simulink model "MPC_System"  (R2019a)
settings: Solver=VariableStepAuto  StartTime=0.0  StopTime=20  RelTol=1e-3
libraries: sailbot_library x19, mpclib x1
settings Model: Creator=ronak  LastModifiedBy=brucecui
settings DataIOCC: SaveFormat=StructureWithTime

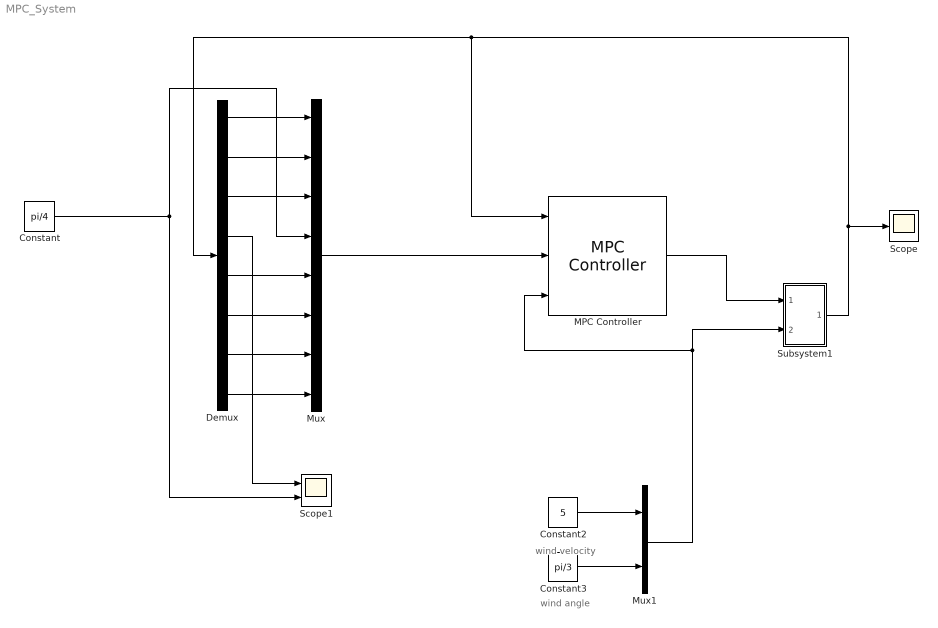
== system MPC_System ==
  note: wind velocity
  note: wind angle
  Constant : Constant  Value=pi/4
  Constant2 : Constant  Value=5
  Constant3 : Constant  Value=pi/3
  Demux : Demux  Outputs=8
  MPC Controller : mpclib/MPC Controller  SCDEnableBlockLinearizationSpecification=on  mpcobj=mpc1  is_multiple=0  enable_value=0  return_u0=off  updateMPCinCallerWorkspace=on  md_inport=on  mv_inport=off  uref_inport=off  return_cost=off  return_mvseq=off  return_qpstatus=off  return_xseq=off  return_state=off  return_ovseq=off  state_inport=off  umin_inport=off  umax_inport=off  ymin_inport=off  ymax_inport=off  cc_inport=off  ywt_inport=off  uwt_inport=off  duwt_inport=off  rhoeps_inport=off  pm_inport=off  MaximumP=10  HorizonChoice=FixedHorizon  n_ts=1  n_p=10  n_mv=2  n_md=2  n_ud=0  n_mo=8  n_uo=0  BlockDataType=double  SampleTimeInherited=off  switch_inport=off
      settings: SourceProductName=MATLAB Runtime - Model Predictive Control Toolbox Addin  SourceProductBaseCode=Missing
  Mux : Mux  Inputs=8
  Mux1 : Mux  Inputs=2
  Scope : Scope
  Scope1 : Scope  NumInputPorts=2
  Subsystem1 : Subsystem
  wires:
  Constant2/1 -> Mux1/1
  Demux/1 -> Mux/1
  Demux/2 -> Mux/2
  Demux/7 -> Mux/7
  Demux/3 -> Mux/3
  MPC Controller/1 -> Subsystem1/1(In1)
  Demux/8 -> Mux/8
  Demux/5 -> Mux/5
  Constant/1 -> Scope1/2, Mux/4
  Constant3/1 -> Mux1/2
  Demux/4 -> Scope1/1
  Demux/6 -> Mux/6
  Mux/1 -> MPC Controller/2
  Subsystem1/1(Out2) -> Scope/1, MPC Controller/1, Demux/1
  Mux1/1 -> MPC Controller/3, Subsystem1/2(In2)

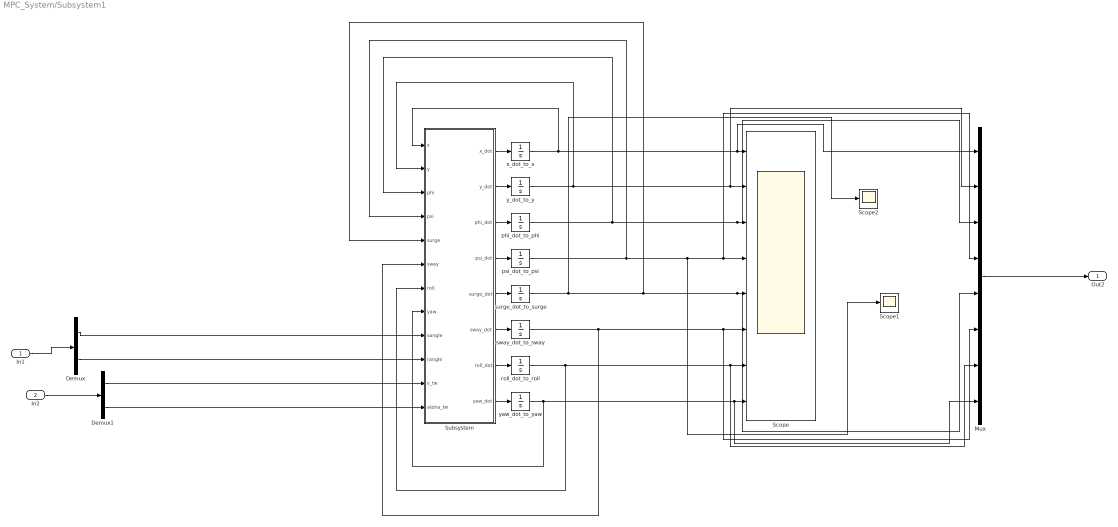
== system MPC_System/Subsystem1 ==
  In1 : Inport
  In2 : Inport  Port=2
  Demux : Demux  Outputs=2
  Demux1 : Demux  Outputs=2
  Mux : Mux  Inputs=8
  Scope : Scope  NumInputPorts=8
  Scope1 : Scope
  Scope2 : Scope
  Subsystem : Subsystem
  phi_dot_to_phi : Integrator  InitialCondition=0.05
  psi_dot_to_psi : Integrator  InitialCondition=0.05
  roll_dot_to_roll : Integrator  InitialCondition=0.05
  surge_dot_to_surge : Integrator  InitialCondition=0.05
  sway_dot_to_sway : Integrator  InitialCondition=0.05
  x_dot_to_x : Integrator  InitialCondition=0.05
  y_dot_to_y : Integrator  InitialCondition=0.05
  yaw_dot_to_yaw : Integrator  InitialCondition=0.05
  Out2 : Outport
  wires:
  x_dot_to_x/1 -> Mux/1, Scope/1, Subsystem/1(x)
  y_dot_to_y/1 -> Scope/2, Mux/2, Subsystem/2(y)
  phi_dot_to_phi/1 -> Subsystem/3(phi), Mux/3, Scope/3
  sway_dot_to_sway/1 -> Scope/6, Mux/6, Subsystem/6(sway)
  Subsystem/5(surge_dot) -> surge_dot_to_surge/1
  yaw_dot_to_yaw/1 -> Scope/8, Mux/8, Subsystem/8(yaw)
  roll_dot_to_roll/1 -> Scope/7, Mux/7, Subsystem/7(roll)
  psi_dot_to_psi/1 -> Subsystem/4(psi), Scope1/1, Scope/4, Mux/4
  Subsystem/1(x_dot) -> x_dot_to_x/1
  surge_dot_to_surge/1 -> Scope2/1, Subsystem/5(surge), Mux/5, Scope/5
  Subsystem/8(yaw_dot) -> yaw_dot_to_yaw/1
  Subsystem/4(psi_dot) -> psi_dot_to_psi/1
  Subsystem/3(phi_dot) -> phi_dot_to_phi/1
  Subsystem/6(sway_dot) -> sway_dot_to_sway/1
  Subsystem/2(y_dot) -> y_dot_to_y/1
  Subsystem/7(roll_dot) -> roll_dot_to_roll/1
  Mux/1 -> Out2/1
  Demux/1 -> Subsystem/9(sangle)
  Demux/2 -> Subsystem/10(rangle)
  In1/1 -> Demux/1
  Demux1/1 -> Subsystem/11(v_tw)
  Demux1/2 -> Subsystem/12(alpha_tw)
  In2/1 -> Demux1/1

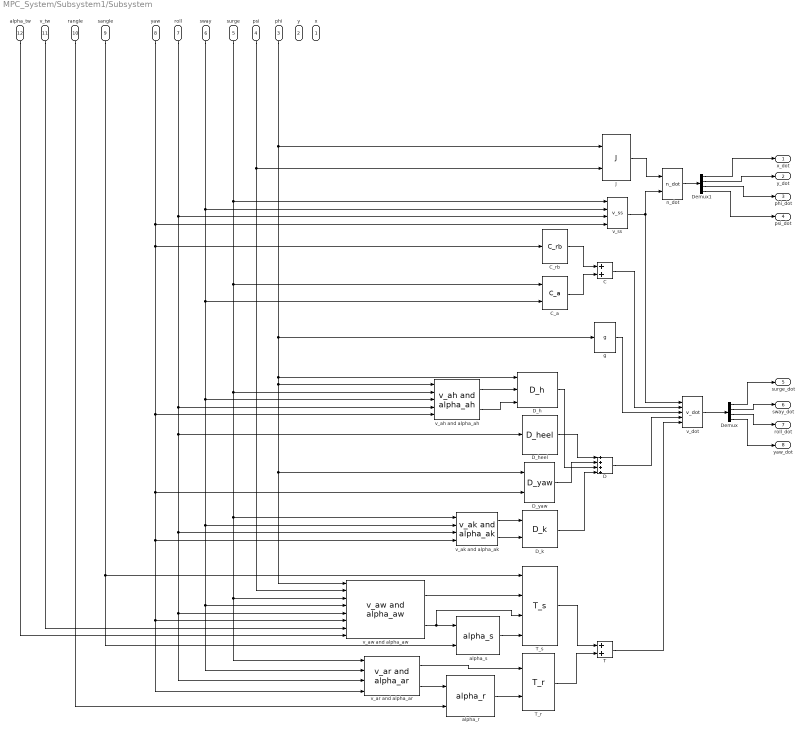
== system MPC_System/Subsystem1/Subsystem ==
  x : Inport
  y : Inport  Port=2
  phi : Inport  Port=3
  psi : Inport  Port=4
  surge : Inport  Port=5
  sway : Inport  Port=6
  roll : Inport  Port=7
  yaw : Inport  Port=8
  sangle : Inport  Port=9
  rangle : Inport  Port=10
  v_tw : Inport  Port=11
  alpha_tw : Inport  Port=12
  C : Sum
  C_a : sailbot_library/C_a  SystemSampleTime=-1
  C_rb : sailbot_library/C_rb  SystemSampleTime=-1
  D : Sum  Inputs=4
  D_h : sailbot_library/D_h  SystemSampleTime=-1
  "D_heel " : sailbot_library/D_heel   SystemSampleTime=-1
  D_k : sailbot_library/D_k  SystemSampleTime=-1
  D_yaw : sailbot_library/D_yaw  SystemSampleTime=-1
  Demux : Demux
  Demux1 : Demux
  J : sailbot_library/J  SystemSampleTime=-1
  T : Sum
  T_r : sailbot_library/T_r  SystemSampleTime=-1
  "T_s " : sailbot_library/T_s   SystemSampleTime=-1
  alpha_r : sailbot_library/alpha_r  SystemSampleTime=-1
  alpha_s : sailbot_library/alpha_s  SystemSampleTime=-1
  g : sailbot_library/g  SystemSampleTime=-1
  n_dot : sailbot_library/n_dot  SystemSampleTime=-1
  v_ah and alpha_ah : sailbot_library/v_ah and alpha_ah  SystemSampleTime=-1
  v_ak and alpha_ak : sailbot_library/v_ak and alpha_ak  SystemSampleTime=-1
  v_ar and alpha_ar : sailbot_library/v_ar and alpha_ar  SystemSampleTime=-1
  v_aw and alpha_aw : sailbot_library/v_aw and alpha_aw  SystemSampleTime=-1
  v_dot : sailbot_library/v_dot  SystemSampleTime=-1
  v_ss : sailbot_library/v_ss  SystemSampleTime=-1
  x_dot : Outport
  y_dot : Outport  Port=2
  phi_dot : Outport  Port=3
  psi_dot : Outport  Port=4
  surge_dot : Outport  Port=5
  sway_dot : Outport  Port=6
  roll_dot : Outport  Port=7
  yaw_dot : Outport  Port=8
  wires:
  alpha_s/1 -> "T_s "/4
  Demux/4 -> yaw_dot/1
  C/1 -> v_dot/2
  v_ah and alpha_ah/1 -> D_h/2
  D/1 -> v_dot/4
  v_aw and alpha_aw/1 -> "T_s "/2
  v_ak and alpha_ak/1 -> D_k/1
  v_ak and alpha_ak/2 -> D_k/2
  Demux/3 -> roll_dot/1
  C_a/1 -> C/2
  J/1 -> n_dot/1
  psi/1 -> v_aw and alpha_aw/2, J/2
  Demux1/4 -> psi_dot/1
  Demux1/2 -> y_dot/1
  T/1 -> v_dot/5
  v_aw and alpha_aw/2 -> "T_s "/3, alpha_s/1
  alpha_tw/1 -> v_aw and alpha_aw/8
  sway/1 -> v_ss/2, C_a/2, v_ah and alpha_ah/3, v_aw and alpha_aw/4, v_ar and alpha_ar/2, v_ak and alpha_ak/2
  alpha_r/1 -> T_r/2
  v_tw/1 -> v_aw and alpha_aw/7
  g/1 -> v_dot/3
  C_rb/1 -> C/1
  v_ah and alpha_ah/2 -> D_h/3
  v_ss/1 -> v_dot/1, n_dot/2
  n_dot/1 -> Demux1/1
  Demux1/3 -> phi_dot/1
  surge/1 -> v_ak and alpha_ak/1, v_aw and alpha_aw/3, v_ar and alpha_ar/1, v_ah and alpha_ah/2, C_a/1, v_ss/1
  Demux1/1 -> x_dot/1
  v_ar and alpha_ar/1 -> T_r/1
  rangle/1 -> alpha_r/2
  yaw/1 -> v_ss/4, D_yaw/2, v_ak and alpha_ak/4, v_ar and alpha_ar/4, v_aw and alpha_aw/6, v_ah and alpha_ah/5, C_rb/1
  phi/1 -> J/1, D_h/1, D_yaw/1, v_aw and alpha_aw/1, v_ah and alpha_ah/1, g/1
  Demux/1 -> surge_dot/1
  sangle/1 -> "T_s "/1, alpha_s/2
  v_ar and alpha_ar/2 -> alpha_r/1
  Demux/2 -> sway_dot/1
  roll/1 -> v_ss/3, v_ah and alpha_ah/4, "D_heel "/1, v_ak and alpha_ak/3, v_aw and alpha_aw/5, v_ar and alpha_ar/3
  v_dot/1 -> Demux/1
  "D_heel "/1 -> D/1
  D_yaw/1 -> D/2
  D_h/1 -> D/3
  D_k/1 -> D/4
  T_r/1 -> T/2
  "T_s "/1 -> T/1
